simulink model "modelo_stateflow"  (R2023a)
settings: Solver=VariableStepAuto  StartTime=0.0  StopTime=10.0  RelTol=1e-3
InitFcn:
  | w_hm_min_BRK = 999999;
  | w_tm_min_BRK = 999999;
settings Model: PacingRate=0.630000  Creator=Usuario  LastModifiedBy=Usuario

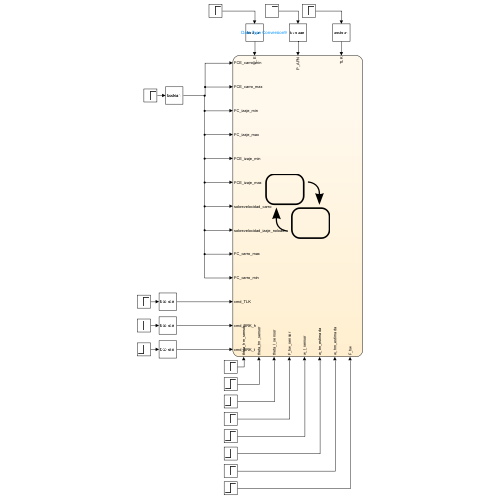
[thumbnail: Simulink's stored preview of the top-level diagram]
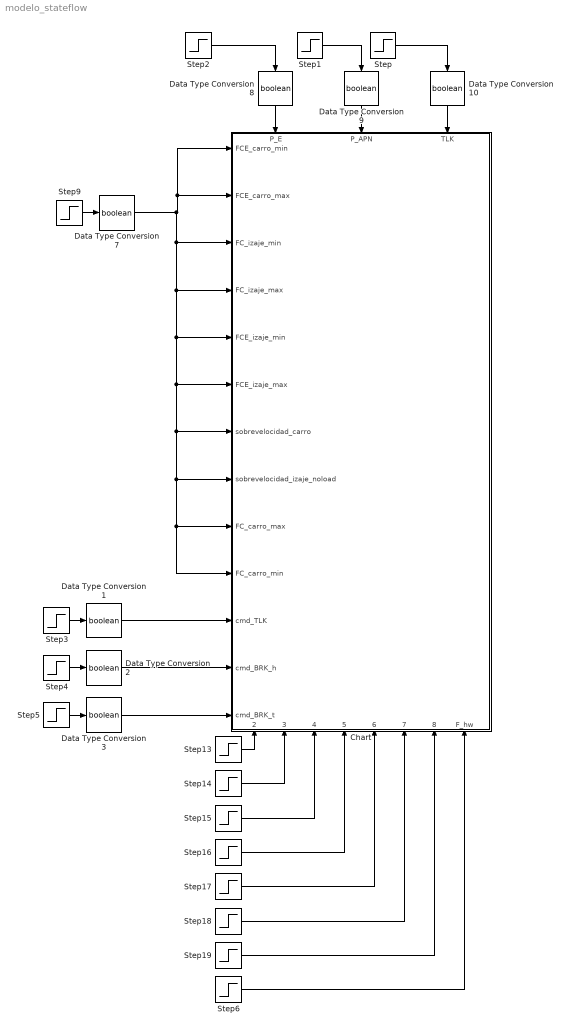
== system modelo_stateflow ==
  Chart : Stateflow chart  TreatAsAtomicUnit=on
      settings: PortSchema="{\"entries\":[{\"content\":{\"sides\":[{\"content\":{\"connectorIds\":[\"In11\",\"In12\",\"In13\",\"In14\",\"In15\",\"In16\",\"In17\",\"In18\",\"In19\",\"In20\",\"In21\",\"In22\",\"In23\"]},\"type\":\"ConnectorPlacement.EquallySpacedRectSide\",\"uuid\":\"7880b9cd-08fb-4733-bb6b-48e405180dc5\"},{\"content\":{\"side\":\"RIGHT\"},\"type\":\"ConnectorPlacement.EquallySpacedRectSide\",\"uuid\":\"1a0088c7-0ec1-46fb-bd67-3069194311ce\"},{\"content\":{\"connectorIds\":[\"In10\",\"In9\",\"In1\"],\"side\":\"TOP\"},\"type\":\"ConnectorPlacement.EquallySpacedRectSide\",\"uuid\":\"63c24ea1-9c7d-47d6-85d5-bbef0a7be167\"},{\"content\":{\"connectorIds\":[\"In2\",\"In3\",\"In4\",\"In5\",\"In6\",\"In7\",\"In8\",\"In24\"],\"side\":\"BOTTOM\"},\"type\":\"ConnectorPlacement.EquallySpacedRectSide\",\"uuid\":\"56586e70-7155-4caa-800e-4bb67e399bfa\"}]},\"type\":\"ConnectorPlacement.EquallySpacedConnector\",\"uuid\":\"e7da0abc-eae0-41d9-ad4b-a3df1daa3702\"}],\"packageUris\":[\"http://schema.mathworks.com/mf0/Connector/R2020b\"],\"version\":\"1.0\"}"
  Data Type Conversion{1..3,7..10} (7 alike) : DataTypeConversion  OutDataTypeStr=boolean  SaturateOnIntegerOverflow=off  RndMeth=Floor
  Step{,2,4..6,9,13..19} (13 alike) : Step  After=0  SampleTime=0
  Step1 : Step  Time=5  SampleTime=0
  Step3 : Step  Time=5  After=0  SampleTime=0
  wires:
  Step/1 -> Data Type Conversion10/1
  Step1/1 -> Data Type Conversion9/1
  Step2/1 -> Data Type Conversion8/1
  Step13/1 -> Chart/2(theta_hm_sensor)
  Step14/1 -> Chart/3(theta_tm_sensor)
  Step15/1 -> Chart/4(theta_l_sensor)
  Step16/1 -> Chart/5(F_hw_sensor)
  Step17/1 -> Chart/6(w_l_sensor)
  Step18/1 -> Chart/7(w_tm_estimada)
  Step19/1 -> Chart/8(w_hm_estimada)
  Step9/1 -> Data Type Conversion7/1
  Data Type Conversion8/1 -> Chart/10(P_E)
  Data Type Conversion9/1 -> Chart/9(P_APN)
  Data Type Conversion10/1 -> Chart/1(TLK)
  Data Type Conversion7/1 -> Chart/16(FCE_izaje_max), Chart/17(sobrevelocidad_carro), Chart/19(FC_carro_max), Chart/20(FC_carro_min), Chart/18(sobrevelocidad_izaje_noload), Chart/15(FCE_izaje_min), Chart/14(FC_izaje_max), Chart/13(FC_izaje_min), Chart/12(FCE_carro_max), Chart/11(FCE_carro_min)
  Step3/1 -> Data Type Conversion1/1
  Data Type Conversion1/1 -> Chart/21(cmd_TLK)
  Step4/1 -> Data Type Conversion2/1
  Data Type Conversion2/1 -> Chart/22(cmd_BRK_h)
  Step5/1 -> Data Type Conversion3/1
  Data Type Conversion3/1 -> Chart/23(cmd_BRK_t)
  Step6/1 -> Chart/24(F_hw)

== stateflow chart modelo_stateflow/Chart ==
  state Nivel 1 - Control Supervisor
    state ON
      state BRK_Logic [parallel]
        settings: executionOrder=1
        state BRK_t_Logic [parallel]
          settings: executionOrder=1
          state BRK_t_Closed
          state BRK_t_Opened
          (default) -> BRK_t_Closed
          BRK_t_Opened -> BRK_t_Closed : [(rising(cmd_BRK_t) && abs(w_tm_estimada) < w_tm_min_BRK) || FC_carro_min || FC_carro_max]
          BRK_t_Closed -> BRK_t_Opened : [falling(cmd_BRK_t) && ~(FC_carro_max || FC_carro_min)]
        state BRK_h_Logic [parallel]
          settings: executionOrder=2
          state BRK_h_Closed
          state BRK_h_Opened
          (default) -> BRK_h_Closed
          BRK_h_Opened -> BRK_h_Closed : [(rising(cmd_BRK_h) && abs(w_hm_estimada) < w_hm_min_BRK) || FC_izaje_min || FC_izaje_max]
          BRK_h_Closed -> BRK_h_Opened : [falling(cmd_BRK_h) && ~(FC_izaje_max || FC_izaje_min)]
      state TLK_Logic [parallel]
        settings: executionOrder=2
        state Init
        state TLK_Opened
        state TLK_Closed
        (default) -> Init
        Init -> TLK_Opened [order 2] : [~cmd_TLK]
        Init -> TLK_Closed [order 1] : [cmd_TLK]
        TLK_Opened -> TLK_Closed : [rising(cmd_TLK) && abs(F_hw) <= 10]
        TLK_Closed -> TLK_Opened : [falling(cmd_TLK) && abs(F_hw) <= 10]
    state OFF
    (default) -> OFF
    OFF -> ON : [rising(P_APN)]
    ON -> OFF : [falling(P_APN)]
  (default) -> Nivel 1 - Control Supervisor
  data: TLK input; theta_hm_sensor input; theta_tm_sensor input; theta_l_sensor input; F_hw_sensor input; w_l_sensor input; w_tm_estimada input; w_hm_estimada input; P_APN input; P_E input; FCE_carro_min input; FCE_carro_max input; FC_izaje_min input; FC_izaje_max input; FCE_izaje_min input; FCE_izaje_max input; sobrevelocidad_carro input; sobrevelocidad_izaje_noload input; FC_carro_max input; FC_carro_min input; cmd_TLK input; cmd_BRK_h input; cmd_BRK_t input; F_hw input; w_hm_min_BRK parameter; w_tm_min_BRK parameter
